simulink model "ROS"  (R2017b)
settings: Solver=FixedStepDiscrete  StartTime=0.0  StopTime=1000  FixedStep=0.01  RelTol=1e-3  EnableMultiTasking=on
libraries: robotlib x6
settings Model: Creator=The MathWorks, Inc.  LastModifiedBy=radian
settings DataIOCC: LimitDataPoints=on  SaveFormat=Array
settings OptimizationCC: LifeSpan=1  MaxStackSize=64
settings DebuggingCC: SolverPrmCheckMsg=warning  SFUnexpectedBacktrackingDiag=warning  SFNoUnconditionalDefaultTransitionDiag=warning  SFExecutionAtInitializationDiag=none
settings HardwareCC: ProdBitPerPointer=32  ProdBitPerSizeT=32  ProdBitPerPtrDiffT=32  ProdLargestAtomicFloat=None  ProdIntDivRoundTo=Undefined  ProdEndianess=Unspecified  ProdWordSize=32  ProdHWDeviceType=Generic->Unspecified (assume 32-bit Generic)  TargetHWDeviceType=Generic->Unspecified (assume 32-bit Generic)  UseEmbeddedCoderFeatures=off
settings ModelReferenceCC: PropagateSignalLabelsOutOfModel=off
settings RTWCC: SystemTargetFile=ert.tlc  HardwareBoard=Robot Operating System (ROS)  TLCOptions=-aInlineSetEventsForThisBaseRateFcn=TLC_FALSE -aSuppressMultiTaskScheduler=TLC_FALSE -aRateBasedStepFcn=0  TemplateMakefile=ert_default_tmf  Toolchain=Catkin  TargetLang=C++
settings CodeAppCC: StateflowObjectComments=on
settings ERTTargetCC: MultiwordLength=2048  ERTCustomFileBanners=off  MultiInstanceERTCode=on  CodeInterfacePackaging=C++ class  SupportContinuousTime=on  SupportNonInlinedSFcns=on  RemoveResetFunc=off  SupportVariableSizeSignals=on  ModelStepFunctionPrototypeControlCompliant=off  RootIOFormat=Structure reference  ConvertIfToSwitch=off  SuppressUnreachableDefaultCases=off
settings ConfigComp: CovMetricSettings=dw  CovHtmlReporting=on  CovSaveCumulativeToWorkspaceVar=on  CovSaveSingleToWorkspaceVar=on  CovExternalEMLEnable=off  CovSFcnEnable=off

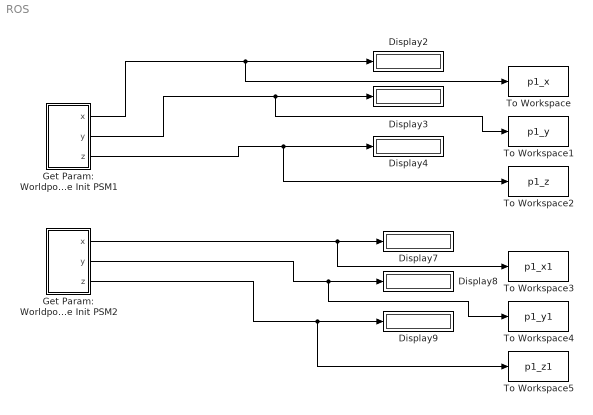
== system ROS ==
  Display{2..4,7..9} (6 alike) : Display
  Get Param: Worldpose Init PSM1 : Subsystem
  Get Param: Worldpose Init PSM2 : Subsystem
  To Workspace : ToWorkspace  VariableName=p1_x  SaveFormat=Timeseries  SampleTime=-1
  To Workspace1 : ToWorkspace  VariableName=p1_y  SaveFormat=Timeseries  SampleTime=-1
  To Workspace2 : ToWorkspace  VariableName=p1_z  SaveFormat=Timeseries  SampleTime=-1
  To Workspace3 : ToWorkspace  VariableName=p1_x1  SaveFormat=Timeseries  SampleTime=-1
  To Workspace4 : ToWorkspace  VariableName=p1_y1  SaveFormat=Timeseries  SampleTime=-1
  To Workspace5 : ToWorkspace  VariableName=p1_z1  SaveFormat=Timeseries  SampleTime=-1
  wires:
  Get Param: Worldpose Init PSM1/1(x) -> To Workspace/1, Display2/1
  Get Param: Worldpose Init PSM1/2(y) -> To Workspace1/1, Display3/1
  Get Param: Worldpose Init PSM1/3(z) -> To Workspace2/1, Display4/1
  Get Param: Worldpose Init PSM2/1(x) -> To Workspace3/1, Display7/1
  Get Param: Worldpose Init PSM2/2(y) -> To Workspace4/1, Display8/1
  Get Param: Worldpose Init PSM2/3(z) -> To Workspace5/1, Display9/1

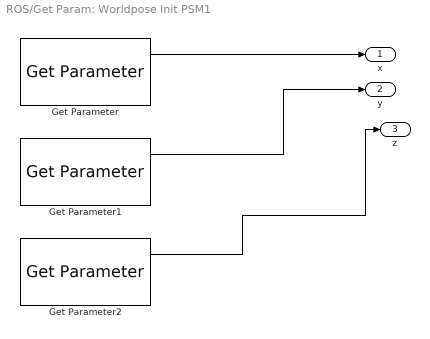
== system ROS/Get Param: Worldpose Init PSM1 ==
  Get Parameter : robotlib/Get Parameter  SourceLibraryInfo=This block requires Robotics System Toolbox  ParameterSource=Specify your own  ParameterName=/one_init_tool/x  ParameterType=double  ParameterMaxArrayLength=16  ParameterInitialValue=0.0  SampleTime=-1  ShowErrorCodeOutput=on  ModelName=ROS  BlockId=ParamGet_ROS_43
      settings: SourceProductName=Robotics System Toolbox  SourceProductBaseCode=RO
  Get Parameter1 : robotlib/Get Parameter  SourceLibraryInfo=This block requires Robotics System Toolbox  ParameterSource=Specify your own  ParameterName=/one_init_tool/y  ParameterType=double  ParameterMaxArrayLength=16  ParameterInitialValue=0.0  SampleTime=-1  ShowErrorCodeOutput=on  ModelName=ROS  BlockId=ParamGet_ROS_50
      settings: SourceProductName=Robotics System Toolbox  SourceProductBaseCode=RO
  Get Parameter2 : robotlib/Get Parameter  SourceLibraryInfo=This block requires Robotics System Toolbox  ParameterSource=Specify your own  ParameterName=/one_init_tool/z  ParameterType=double  ParameterMaxArrayLength=16  ParameterInitialValue=0.0  SampleTime=-1  ShowErrorCodeOutput=on  ModelName=ROS  BlockId=ParamGet_ROS_51
      settings: SourceProductName=Robotics System Toolbox  SourceProductBaseCode=RO
  x : Outport
  y : Outport  Port=2
  z : Outport  Port=3
  wires:
  Get Parameter2/1 -> z/1
  Get Parameter1/1 -> y/1
  Get Parameter/1 -> x/1

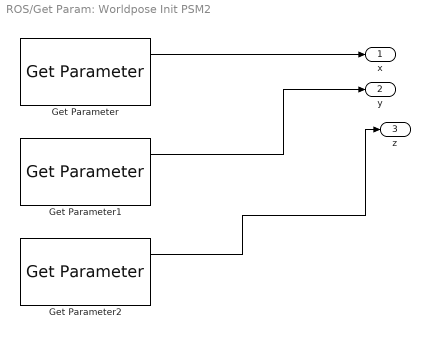
== system ROS/Get Param: Worldpose Init PSM2 ==
  Get Parameter : robotlib/Get Parameter  SourceLibraryInfo=This block requires Robotics System Toolbox  ParameterSource=Specify your own  ParameterName=/two_init_tool/x  ParameterType=double  ParameterMaxArrayLength=16  ParameterInitialValue=0.0  SampleTime=-1  ShowErrorCodeOutput=on  ModelName=ROS  BlockId=ParamGet_ROS_60
      settings: SourceProductName=Robotics System Toolbox  SourceProductBaseCode=RO
  Get Parameter1 : robotlib/Get Parameter  SourceLibraryInfo=This block requires Robotics System Toolbox  ParameterSource=Specify your own  ParameterName=/two_init_tool/y  ParameterType=double  ParameterMaxArrayLength=16  ParameterInitialValue=0.0  SampleTime=-1  ShowErrorCodeOutput=on  ModelName=ROS  BlockId=ParamGet_ROS_61
      settings: SourceProductName=Robotics System Toolbox  SourceProductBaseCode=RO
  Get Parameter2 : robotlib/Get Parameter  SourceLibraryInfo=This block requires Robotics System Toolbox  ParameterSource=Specify your own  ParameterName=/two_init_tool/z  ParameterType=double  ParameterMaxArrayLength=16  ParameterInitialValue=0.0  SampleTime=-1  ShowErrorCodeOutput=on  ModelName=ROS  BlockId=ParamGet_ROS_62
      settings: SourceProductName=Robotics System Toolbox  SourceProductBaseCode=RO
  x : Outport
  y : Outport  Port=2
  z : Outport  Port=3
  wires:
  Get Parameter2/1 -> z/1
  Get Parameter1/1 -> y/1
  Get Parameter/1 -> x/1
